simulink model "crazyflie"  (R2023a)
settings: Solver=FixedStepDiscrete  StartTime=0.0  StopTime=160  FixedStep=0.001  RelTol=1e-3
undefined symbols (not defined in the file or in its folder): DiscIntNeverNeededParam, K
settings Model: PauseTimes=7  Creator=Zrean  LastModifiedBy=anton
settings SolverCC: AlgebraicLoopSolver=TrustRegion
settings DataIOCC: ReturnWorkspaceOutputs=off
settings OptimizationCC: DefaultParameterBehavior=Inlined  UseDivisionForNetSlopeComputation=on  UseFloatMulNetSlope=on  UseSpecifiedMinMax=on  InlineInvariantSignals=on  PassReuseOutputArgsAs=Individual arguments  ZeroExternalMemoryAtStartup=off  ZeroInternalMemoryAtStartup=off  NoFixptDivByZeroProtection=on  EfficientFloat2IntCast=on  LifeSpan=1  EfficientTunableParamExpr=on
settings DebuggingCC: AlgebraicLoopMsg=error  ParameterTunabilityLossMsg=error  UnconnectedInputMsg=warning  UnconnectedOutputMsg=warning  UnconnectedLineMsg=warning  ArithmeticOperatorsInVariantConditions=warning
settings HardwareCC: ProdBitPerPointer=32  ProdBitPerSizeT=32  ProdBitPerPtrDiffT=32  ProdLargestAtomicInteger=Long  ProdLargestAtomicFloat=Double  ProdWordSize=32  ProdHWDeviceType=ARM Compatible->ARM Cortex
settings ModelReferenceCC: EnableRefExpFcnMdlSchedulingChecks=on
settings SFSimCC: SimUseLocalCustomCode=off  MATLABDynamicMemAlloc=off  CustomCodeUndefinedFunction=UseInterfaceOnly
settings RTWCC: Description=Embedded Coder  SystemTargetFile=ert.tlc  GenCodeOnly=on  TemplateMakefile=ert_default_tmf  GenerateReport=on  RTWUseLocalCustomCode=off  BuildConfiguration=Faster Runs  IncludeHyperlinkInReport=on  LaunchReport=on  GenerateTraceInfo=on  GenerateTraceReport=on  GenerateTraceReportSl=on  GenerateTraceReportSf=on  GenerateTraceReportEml=on  GenerateCodeMetricsReport=on
settings CodeAppCC: ForceParamTrailComments=on  IgnoreCustomStorageClasses=off  OperatorAnnotations=on  SimulinkDataObjDesc=on  SFDataObjDesc=on  MATLABFcnDesc=on  InsertBlockDesc=on  StateflowObjectComments=on  MATLABSourceComments=on
settings ERTTargetCC: TargetLangStandard=C99 (ISO)  MultiwordLength=2048  CombineSignalStateStructs=on  SuppressErrorStatus=on  SupportAbsoluteTime=off  SupportNonFinite=off  SupportComplex=off  InlinedParameterPlacement=NonHierarchical  ERTCustomFileTemplate=crazyflie_wrapper.tlc  ERTFilePackagingFormat=CompactWithDataFile
settings SimscapeCC: SimscapeNormalizeSystem=off

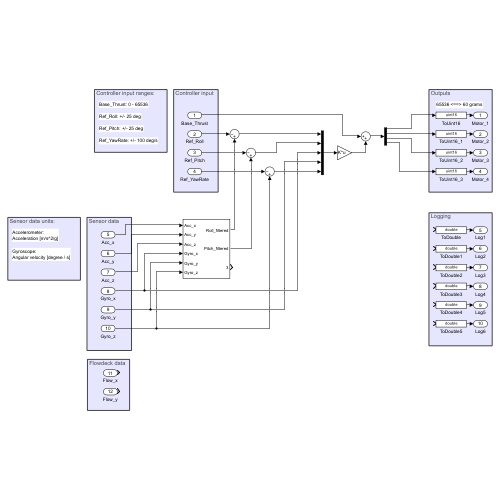
[thumbnail: Simulink's stored preview of the top-level diagram]
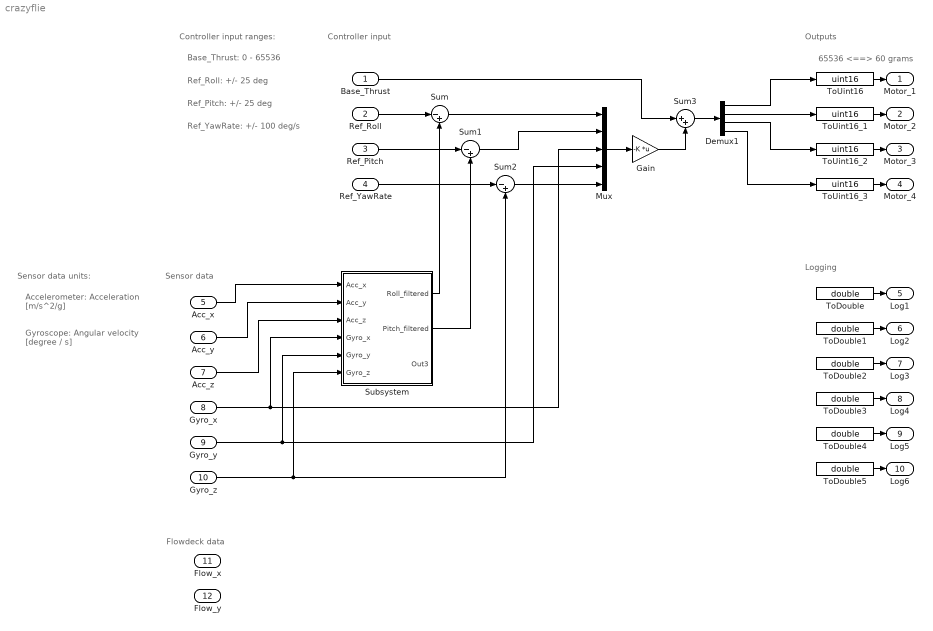
== system crazyflie ==
  note: 65536 <==> 60 grams
  note: Logging
  note: Outputs
  note: Sensor data
  note: Controller input
  note: Ref_Roll: +/- 25 deg
  note: Base_Thrust: 0 - 65536
  note: Ref_Pitch: +/- 25 deg
  note: Ref_YawRate: +/- 100 deg/s
  note: Controller input ranges:
  note: Gyroscope:
      | Angular velocity [degree / s]
  note: Accelerometer:
      | Acceleration [m/s^2/g]
  note: Sensor data units:
  note: Flowdeck data
  Base_Thrust : Inport  OutDataTypeStr=double
  Ref_Roll : Inport  Port=2  OutDataTypeStr=double
  Ref_Pitch : Inport  Port=3  OutDataTypeStr=double
  Ref_YawRate : Inport  Port=4  OutDataTypeStr=double
  Acc_x : Inport  Port=5  OutDataTypeStr=double  PortDimensions=1
  Acc_y : Inport  Port=6  OutDataTypeStr=double  PortDimensions=1
  Acc_z : Inport  Port=7  OutDataTypeStr=double  PortDimensions=1
  Gyro_x : Inport  Port=8  OutDataTypeStr=double  PortDimensions=1
  Gyro_y : Inport  Port=9  OutDataTypeStr=double  PortDimensions=1
  Gyro_z : Inport  Port=10  OutDataTypeStr=double  PortDimensions=1
  Flow_x : Inport  Port=11  OutDataTypeStr=int16  PortDimensions=1
  Flow_y : Inport  Port=12  OutDataTypeStr=int16  PortDimensions=1
  Demux1 : Demux
  Gain : Gain  Gain=-K  Multiplication=Matrix(K*u)
  Mux : Mux  Inputs=5
  Subsystem : Subsystem
  Sum : Sum  Inputs=|-+
  Sum1 : Sum  Inputs=|-+
  Sum2 : Sum  Inputs=|-+
  Sum3 : Sum  Inputs=|++
  ToDouble{,1..5} (6 alike) : DataTypeConversion  OutDataTypeStr=double  RndMeth=Floor
  ToUint16 : DataTypeConversion  OutDataTypeStr=uint16  RndMeth=Floor
  ToUint16_1 : DataTypeConversion  OutDataTypeStr=uint16  RndMeth=Floor
  ToUint16_2 : DataTypeConversion  OutDataTypeStr=uint16  RndMeth=Floor
  ToUint16_3 : DataTypeConversion  OutDataTypeStr=uint16  RndMeth=Floor
  Motor_1 : Outport  OutDataTypeStr=uint16  VectorParamsAs1DForOutWhenUnconnected=off  LockScale=on
  Motor_2 : Outport  Port=2  OutDataTypeStr=uint16  VectorParamsAs1DForOutWhenUnconnected=off  LockScale=on
  Motor_3 : Outport  Port=3  OutDataTypeStr=uint16  VectorParamsAs1DForOutWhenUnconnected=off  LockScale=on
  Motor_4 : Outport  Port=4  OutDataTypeStr=uint16  VectorParamsAs1DForOutWhenUnconnected=off  LockScale=on
  Log1 : Outport  Port=5  OutDataTypeStr=double  VectorParamsAs1DForOutWhenUnconnected=off
  Log2 : Outport  Port=6  OutDataTypeStr=double  VectorParamsAs1DForOutWhenUnconnected=off
  Log3 : Outport  Port=7  OutDataTypeStr=double  VectorParamsAs1DForOutWhenUnconnected=off
  Log4 : Outport  Port=8  OutDataTypeStr=double  VectorParamsAs1DForOutWhenUnconnected=off
  Log5 : Outport  Port=9  OutDataTypeStr=double  VectorParamsAs1DForOutWhenUnconnected=off
  Log6 : Outport  Port=10  OutDataTypeStr=double  VectorParamsAs1DForOutWhenUnconnected=off
  wires:
  ToUint16/1 -> Motor_1/1
  ToUint16_1/1 -> Motor_2/1
  ToUint16_2/1 -> Motor_3/1
  ToUint16_3/1 -> Motor_4/1
  ToDouble/1 -> Log1/1
  ToDouble1/1 -> Log2/1
  ToDouble2/1 -> Log3/1
  ToDouble3/1 -> Log4/1
  ToDouble4/1 -> Log5/1
  ToDouble5/1 -> Log6/1
  Acc_x/1 -> Subsystem/1(Acc_x)
  Acc_y/1 -> Subsystem/2(Acc_y)
  Acc_z/1 -> Subsystem/3(Acc_z)
  Gyro_x/1 -> Subsystem/4(Gyro_x), Mux/3
  Gyro_y/1 -> Mux/4, Subsystem/5(Gyro_y)
  Gyro_z/1 -> Subsystem/6(Gyro_z), Sum2/2
  Ref_Roll/1 -> Sum/1
  Ref_Pitch/1 -> Sum1/1
  Subsystem/1(Roll_filtered) -> Sum/2
  Subsystem/2(Pitch_filtered) -> Sum1/2
  Ref_YawRate/1 -> Sum2/1
  Sum/1 -> Mux/1
  Sum2/1 -> Mux/5
  Sum1/1 -> Mux/2
  Mux/1 -> Gain/1
  Gain/1 -> Sum3/2
  Base_Thrust/1 -> Sum3/1
  Sum3/1 -> Demux1/1
  Demux1/1 -> ToUint16/1
  Demux1/2 -> ToUint16_1/1
  Demux1/3 -> ToUint16_2/1
  Demux1/4 -> ToUint16_3/1

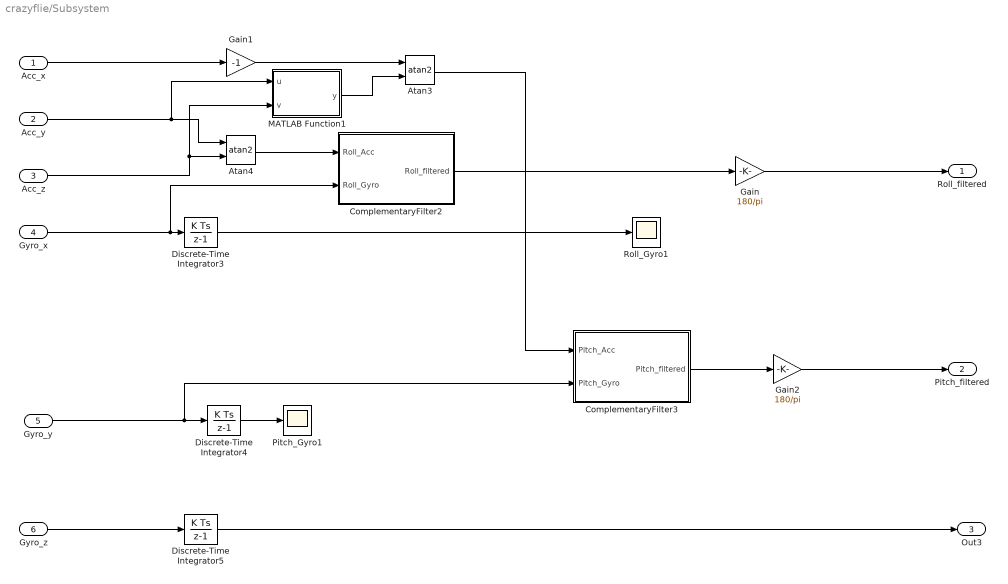
== system crazyflie/Subsystem ==
  Acc_x : Inport
  Acc_y : Inport  Port=2
  Acc_z : Inport  Port=3
  Gyro_x : Inport  Port=4
  Gyro_y : Inport  Port=5
  Gyro_z : Inport  Port=6
  Atan3 : Trigonometry  Operator=atan2
  Atan4 : Trigonometry  Operator=atan2
  ComplementaryFilter2 : Subsystem
  ComplementaryFilter3 : Subsystem
  Discrete-Time Integrator3 : DiscreteIntegrator  gainval=1  SampleTime=0.01  ICPrevOutput=DiscIntNeverNeededParam  ICPrevScaledInput=DiscIntNeverNeededParam
  Discrete-Time Integrator4 : DiscreteIntegrator  gainval=1  SampleTime=0.01  ICPrevOutput=DiscIntNeverNeededParam  ICPrevScaledInput=DiscIntNeverNeededParam
  Discrete-Time Integrator5 : DiscreteIntegrator  gainval=1  SampleTime=0.01  ICPrevOutput=DiscIntNeverNeededParam  ICPrevScaledInput=DiscIntNeverNeededParam
  Gain : Gain  Gain=180/pi
  Gain1 : Gain  Gain=-1
  Gain2 : Gain  Gain=180/pi
  MATLAB Function1 : MATLAB Function  TreatAsAtomicUnit=on
  Pitch_Gyro1 : Scope
  Roll_Gyro1 : Scope
  Roll_filtered : Outport
  Pitch_filtered : Outport  Port=2
  Out3 : Outport  Port=3
  wires:
  Atan3/1 -> ComplementaryFilter3/1(Pitch_Acc)
  Gain1/1 -> Atan3/1
  Gyro_y/1 -> ComplementaryFilter3/2(Pitch_Gyro), Discrete-Time Integrator4/1
  Acc_z/1 -> MATLAB Function1/2(v), Atan4/2
  Discrete-Time Integrator3/1 -> Roll_Gyro1/1
  Gyro_x/1 -> ComplementaryFilter2/2(Roll_Gyro), Discrete-Time Integrator3/1
  MATLAB Function1/1(y) -> Atan3/2
  Atan4/1 -> ComplementaryFilter2/1(Roll_Acc)
  Acc_y/1 -> MATLAB Function1/1(u), Atan4/1
  Discrete-Time Integrator4/1 -> Pitch_Gyro1/1
  Gyro_z/1 -> Discrete-Time Integrator5/1
  Acc_x/1 -> Gain1/1
  Discrete-Time Integrator5/1 -> Out3/1
  ComplementaryFilter2/1(Roll_filtered) -> Gain/1
  ComplementaryFilter3/1(Pitch_filtered) -> Gain2/1
  Gain/1 -> Roll_filtered/1
  Gain2/1 -> Pitch_filtered/1

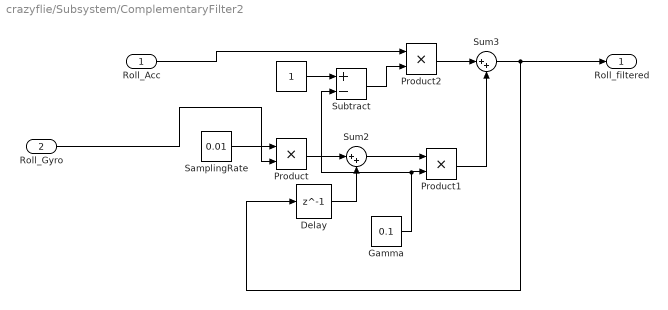
== system crazyflie/Subsystem/ComplementaryFilter2 ==
  Roll_Acc : Inport
  Roll_Gyro : Inport  Port=2
  " " : Constant
  Delay : Delay  DelayLength=1  InitialCondition=0
  Gamma : Constant  Value=0.1
  Product : Product
  Product1 : Product
  Product2 : Product
  SamplingRate : Constant  Value=0.01
  Subtract : Sum  Inputs=+-
  Sum2 : Sum  Inputs=|++
  Sum3 : Sum  Inputs=|++
  Roll_filtered : Outport
  wires:
  Product2/1 -> Sum3/1
  Sum3/1 -> Roll_filtered/1, Delay/1
  Gamma/1 -> Subtract/2, Product1/2
  Sum2/1 -> Product1/1
  Subtract/1 -> Product2/2
  " "/1 -> Subtract/1
  Product/1 -> Sum2/1
  SamplingRate/1 -> Product/1
  Product1/1 -> Sum3/2
  Delay/1 -> Sum2/2
  Roll_Acc/1 -> Product2/1
  Roll_Gyro/1 -> Product/2

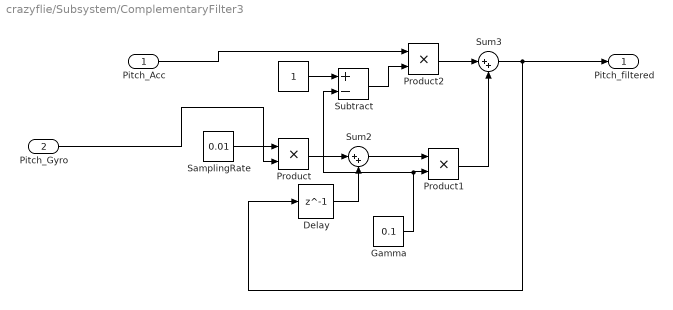
== system crazyflie/Subsystem/ComplementaryFilter3 ==
  Pitch_Acc : Inport
  Pitch_Gyro : Inport  Port=2
  " " : Constant
  Delay : Delay  DelayLength=1  InitialCondition=0
  Gamma : Constant  Value=0.1
  Product : Product
  Product1 : Product
  Product2 : Product
  SamplingRate : Constant  Value=0.01
  Subtract : Sum  Inputs=+-
  Sum2 : Sum  Inputs=|++
  Sum3 : Sum  Inputs=|++
  Pitch_filtered : Outport
  wires:
  Product2/1 -> Sum3/1
  Sum3/1 -> Pitch_filtered/1, Delay/1
  Gamma/1 -> Subtract/2, Product1/2
  Sum2/1 -> Product1/1
  Subtract/1 -> Product2/2
  " "/1 -> Subtract/1
  Product/1 -> Sum2/1
  SamplingRate/1 -> Product/1
  Product1/1 -> Sum3/2
  Delay/1 -> Sum2/2
  Pitch_Acc/1 -> Product2/1
  Pitch_Gyro/1 -> Product/2

== matlab function crazyflie/Subsystem/MATLAB Function1 ==
  data: u input; y output; v input
function y = fcn(u,v)

y = sqrt(u*u+v*v);
end
